simulink model "babv2"  (R2021a)
settings: Solver=VariableStepAuto  StartTime=0.0  StopTime=3000  RelTol=1e-3
libraries: cstblocks x1, dspsrcs4 x1
settings Model: Creator=PC  LastModifiedBy=PC

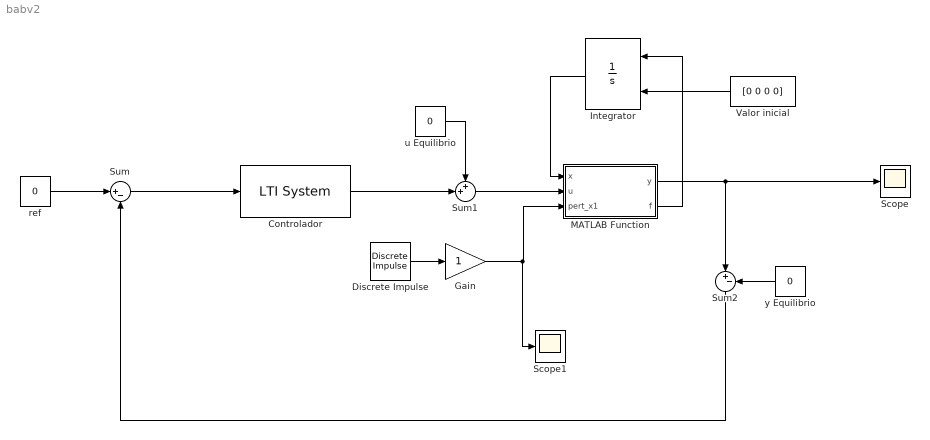
== system babv2 ==
  " ref" : Constant  Value=0
  Controlador : cstblocks/LTI System  sys=0.0002  IC=[]
  Discrete Impulse : dspsrcs4/Discrete  Impulse  Delay=10  SampleTime=1  FrameSample=1  OutputFrames=off  dataType=double  isSigned=on  wordLen=16  udDataType=sfix(16)  fracBitsMode=Best precision  numFracBits=15  OutDataTypeStr=double  LastOutDataTypeStr=double
  Gain : Gain
  Integrator : Integrator  InitialConditionSource=external
  MATLAB Function : MATLAB Function  TreatAsAtomicUnit=on
  Scope : Scope
  Scope1 : Scope
  Sum : Sum  Inputs=|+-
  Sum1 : Sum  Inputs=++|
  Sum2 : Sum  Inputs=|+-
  Valor inicial : Constant  Value=[0 0 0 0]
  u Equilibrio : Constant  Value=0
  y Equilibrio : Constant  Value=0
  wires:
  Valor inicial/1 -> Integrator/2
  Controlador/1 -> Sum1/2
  Sum2/1 -> Sum/2
  y Equilibrio/1 -> Sum2/2
  MATLAB Function/2(f) -> Integrator/1
  MATLAB Function/1(y) -> Scope/1, Sum2/1
  Sum/1 -> Controlador/1
  u Equilibrio/1 -> Sum1/1
  Sum1/1 -> MATLAB Function/2(u)
  Integrator/1 -> MATLAB Function/1(x)
  " ref"/1 -> Sum/1
  Gain/1 -> Scope1/1, MATLAB Function/3(pert_x1)
  Discrete Impulse/1 -> Gain/1

== matlab function babv2/MATLAB Function ==
  data: x input; u input; y output; f output; pert_x1 input
function [y, f] = fcn(x, u, pert_x1)
    
    g = 9.81; %kg m/s2
    m = 0.134; %kg
    kv = 2.1e-3;
    mud = 0.0; 
    mus = 1.6;
    R = 0.02;
    J = 0.5*4*0.007*power(R,2);
    
    x(1) = x(1) + pert_x1;
    
    %Rozamiento estatico
    
    
    %Dinamica
    f1 = x(2);
    f2 = (m*g*sin(x(3)) - kv * x(2) - mud*m*g*cos(x(3)) ) * 1/(m + (J/power(R,2)));
    f3 = x(4);
    f4 = -20.73 * x(4) - 154.47*x(3) + u * 64.89;

    y = x(1);
    f = [f1 f2 f3 f4];
end
